simulink model "test_motion_controller"  (R2025b)
settings: Solver=FixedStepAuto  StartTime=0.0  StopTime=60  RelTol=1e-3
model workspace (MAT data in the model file):
  AmcbldcInitConf = Simulink.Parameter
  AmcbldcInitConf.Value.thresholds.jntVelMax = 40000
  AmcbldcInitConf.Value.thresholds.motorNominalCurrents = 0.34999999404
  AmcbldcInitConf.Value.thresholds.motorPeakCurrents = 0.699999988079
  AmcbldcInitConf.Value.thresholds.motorOverloadCurrents = 1
  AmcbldcInitConf.Value.thresholds.motorPwmLimit = 32000
  AmcbldcInitConf.Value.thresholds.motorCriticalTemperature = 0
  AmcbldcInitConf.Value.pids.currentPID.type : enumeration (value not decoded)
  AmcbldcInitConf.Value.pids.currentPID.OutMax = 0
  AmcbldcInitConf.Value.pids.currentPID.OutMin = 0
  AmcbldcInitConf.Value.pids.currentPID.P = 2
  AmcbldcInitConf.Value.pids.currentPID.I = 500
  AmcbldcInitConf.Value.pids.currentPID.D = 0
  AmcbldcInitConf.Value.pids.currentPID.N = 10
  AmcbldcInitConf.Value.pids.currentPID.I0 = 0
  AmcbldcInitConf.Value.pids.currentPID.D0 = 0
  AmcbldcInitConf.Value.pids.currentPID.shift_factor = 0
  AmcbldcInitConf.Value.pids.velocityPID.type : enumeration (value not decoded)
  AmcbldcInitConf.Value.pids.velocityPID.OutMax = 0
  AmcbldcInitConf.Value.pids.velocityPID.OutMin = 0
  AmcbldcInitConf.Value.pids.velocityPID.P = -20
  AmcbldcInitConf.Value.pids.velocityPID.I = -20
  AmcbldcInitConf.Value.pids.velocityPID.D = 0
  AmcbldcInitConf.Value.pids.velocityPID.N = 100
  AmcbldcInitConf.Value.pids.velocityPID.I0 = 0
  AmcbldcInitConf.Value.pids.velocityPID.D0 = 0
  AmcbldcInitConf.Value.pids.velocityPID.shift_factor = 10
  AmcbldcInitConf.Value.pids.positionPID.type : enumeration (value not decoded)
  AmcbldcInitConf.Value.pids.positionPID.OutMax = 0
  AmcbldcInitConf.Value.pids.positionPID.OutMin = 0
  AmcbldcInitConf.Value.pids.positionPID.P = 0
  AmcbldcInitConf.Value.pids.positionPID.I = 0
  AmcbldcInitConf.Value.pids.positionPID.D = 0
  AmcbldcInitConf.Value.pids.positionPID.N = 0
  AmcbldcInitConf.Value.pids.positionPID.I0 = 0
  AmcbldcInitConf.Value.pids.positionPID.D0 = 0
  AmcbldcInitConf.Value.pids.positionPID.shift_factor = 0
  AmcbldcInitConf.Value.motor.externals.enable_verbosity = 0
  AmcbldcInitConf.Value.motor.externals.has_hall_sens = 1
  AmcbldcInitConf.Value.motor.externals.has_quadrature_encoder = 0
  AmcbldcInitConf.Value.motor.externals.has_speed_quadrature_encoder = 0
  AmcbldcInitConf.Value.motor.externals.has_temperature_sens = 0
  AmcbldcInitConf.Value.motor.externals.encoder_tolerance = 0
  AmcbldcInitConf.Value.motor.externals.pole_pairs = 7
  AmcbldcInitConf.Value.motor.externals.rotor_encoder_resolution = 0
  AmcbldcInitConf.Value.motor.externals.rotor_index_offset = 0
  AmcbldcInitConf.Value.motor.externals.use_index = 0
  AmcbldcInitConf.Value.motor.Kbemf = 0
  AmcbldcInitConf.Value.motor.Rphase = 0
  AmcbldcInitConf.Value.motor.Imin = 0
  AmcbldcInitConf.Value.motor.Imax = 0
  AmcbldcInitConf.Value.motor.Vmax = 24
  AmcbldcInitConf.Value.motor.resistance = 25.8999996185
  AmcbldcInitConf.Value.motor.inductance = 271
  AmcbldcInitConf.Value.motor.thermal_resistance = 16
  AmcbldcInitConf.Value.motor.thermal_time_constant = 797.5
  AmcbldcInitConf.Value.motor.hall_sensors_offset = 30
  AmcbldcInitConf.Value.motor.hall_sensors_swapBC = 0
  AmcbldcInitConf.Value.motor.reference_encoder : enumeration (value not decoded)
  AmcbldcInitConf.Complexity = 'real'
  AmcbldcInitConf.Dimensions = [1 1]
  AmcbldcInitConf.CoderInfo.StorageClass = 'ExportedGlobal'
  AmcbldcInitConf.CoderInfo.Alias = 'AmcbldcInitConf'
  AmcbldcInitConf.DataType = 'Bus: ActuatorConfiguration'
undefined symbols (not defined in the file): ControlModes, EventTypes, MCMotorParamsSet
settings Model: DataDictionary=embeddedBoard_common.sldd  Creator=mfussi  LastModifiedBy=mfussi
settings SolverCC: ConcurrentTasks=on  AutoInsertRateTranBlk=on
settings DataIOCC: SaveOutput=off  DSMLogging=off  SaveTime=off
settings OptimizationCC: DefaultParameterBehavior=Inlined  EnhancedBackFolding=on  PassReuseOutputArgsAs=Individual arguments  ZeroExternalMemoryAtStartup=off  ZeroInternalMemoryAtStartup=off  SimCompilerOptimization=on  OptimizeBlockOrder=speed  DifferentSizesBufferReuse=on  OptimizationCustomize=off  EfficientTunableParamExpr=on
settings DebuggingCC: ParameterPrecisionLossMsg=none  ParameterTunabilityLossMsg=error
settings ModelReferenceCC: SupportModelReferenceSimTargetCustomCode=on
settings SFSimCC: MATLABDynamicMemAlloc=off  SimTargetLang=C++  SimDLTargetLibrary=mkl-dnn
settings RTWCC: SystemTargetFile=ert.tlc  TemplateMakefile=ert_default_tmf  GPUComputeCapability=3.5  Description=Embedded Coder
settings CodeAppCC: ForceParamTrailComments=on  IgnoreCustomStorageClasses=off  MaxIdLength=95.0  OperatorAnnotations=on  SimulinkDataObjDesc=on  SFDataObjDesc=on  InsertBlockDesc=on
settings ERTTargetCC: ERTCustomFileTemplate=example_file_process.tlc  TargetLangStandard=C99 (ISO)  GenerateSampleERTMain=on

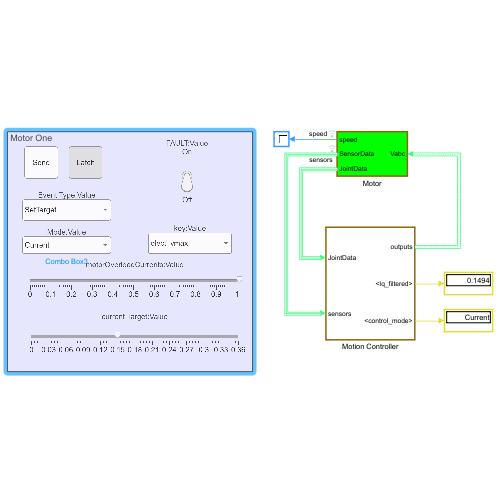
[thumbnail: Simulink's stored preview of the top-level diagram]
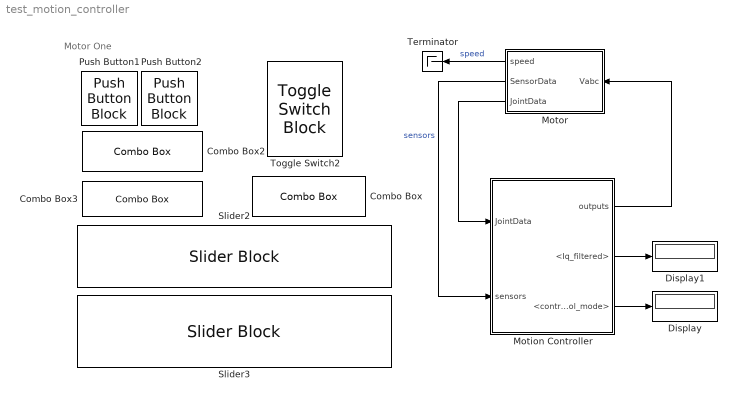
== system test_motion_controller ==
  note: Motor One
  Combo Box : ComboBox  SelectedLabel=elect_vmax  UseEnumeratedDataType=on  EnumeratedDataType=MCMotorParamsSet
  Combo Box2 : ComboBox  SelectedLabel=SetTarget  UseEnumeratedDataType=on  EnumeratedDataType=EventTypes
  Combo Box3 : ComboBox  SelectedLabel=Current  UseEnumeratedDataType=on  EnumeratedDataType=ControlModes
  Display : Display
  Display1 : Display
  Motion Controller : Subsystem
  Motor : Subsystem
  Push Button1 : PushButtonBlock  ButtonText=Send  IconOnColor=[0.0, 0.39215686274509803, 0.0]  IconOffColor=[0.0, 1.0, 0.0]  OffValue=0.000000
  Push Button2 : PushButtonBlock  ButtonText=Latch  ButtonType=Latch  IconOnColor=[0.0, 0.39215686274509803, 0.0]  IconOffColor=[0.0, 1.0, 0.0]  OffValue=0.000000
  Slider2 : SliderBlock  ScaleMax=1
  Slider3 : SliderBlock  ScaleMax=0.36
  Terminator : Terminator
  Toggle Switch2 : ToggleSwitchBlock
  wires:
  Motor/1(speed) -> Terminator/1  "speed"
  Motor/2(SensorData) -> Motion Controller/2(sensors)  "sensors"
  Motor/3(JointData) -> Motion Controller/1(JointData)
  Motion Controller/1(outputs) -> Motor/1(Vabc)
  Motion Controller/2(<Iq_filtered>) -> Display1/1
  Motion Controller/3(<control_mode>) -> Display/1

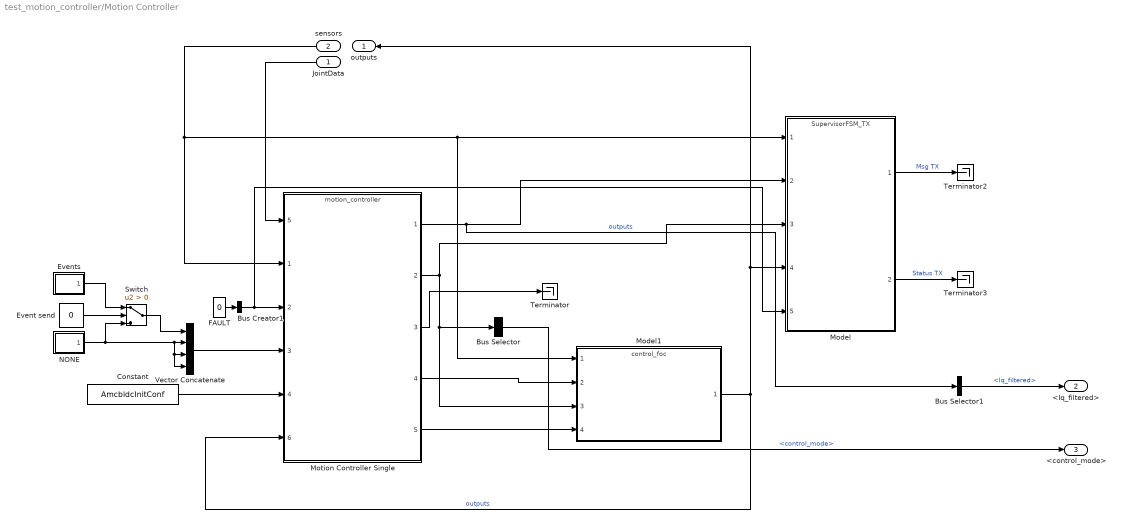
== system test_motion_controller/Motion Controller ==
  JointData : Inport
  sensors : Inport  Port=2
  Bus Creator1 : BusCreator  Inputs=1  OutDataTypeStr=Bus: ExternalFlags  NonVirtualBus=on
      settings: InheritFromInputs=off
  Bus Selector : BusSelector  OutputSignals=control_mode
  Bus Selector1 : BusSelector  OutputSignals=Iq_filtered
  Constant : Constant  Value=AmcbldcInitConf  OutDataTypeStr=Bus: ActuatorConfiguration  SampleTime=1e-3
  Event send : Constant  Value=0  OutDataTypeStr=boolean  SampleTime=1e-3
  Events : Subsystem
  FAULT : Constant  Value=0  OutDataTypeStr=Inherit: Inherit via back propagation  SampleTime=0.001
  Model : ModelReference  ModelNameDialog=SupervisorFSM_TX.slx  SimulationMode=Normal  ModelReferenceVersion=11.18
  Model1 : ModelReference  ModelNameDialog=control_foc.slx  SimulationMode=Normal  ModelReferenceVersion=10.10
  Motion Controller Single : ModelReference  ModelNameDialog=motion_controller.slx  ModelReferenceVersion=6.14
      settings: PortSchema="{\"entries\":[{\"content\":{\"sides\":[{\"content\":{\"connectorIds\":[\"In5\",\"In1\",\"In2\",\"In3\",\"In4\",\"In6\"]},\"type\":\"ConnectorPlacement.EquallySpacedRectSide\",\"uuid\":\"3236986d-16bb-4c67-8dea-b6bfcbd43a75\"},{\"content\":{\"connectorIds\":[\"Out1\",\"Out2\",\"Out3\",\"Out4\",\"Out5\"],\"side\":\"RIGHT\"},\"type\":\"ConnectorPlacement.EquallySpacedRectSide\",\"uuid\":\"7377f631-7d64-4109-b716-f3a651661c1a\"},{\"content\":{\"side\":\"TOP\"},\"type\":\"ConnectorPlacement.EquallySpacedRectSide\",\"uuid\":\"dfb06a46-8687-4228-b411-547df7d03d54\"}]},\"type\":\"ConnectorPlacement.EquallySpacedConnector\",\"uuid\":\"7aeaa35f-2805-4a8c-90e3-68b95f5da4bc\"}],\"packageUris\":[\"http://schema.mathworks.com/mf0/Connector/R2020b\"],\"version\":\"1.0\"}"
  NONE : Subsystem
  Switch : Switch  Criteria=u2 > Threshold  SaturateOnIntegerOverflow=off  InputSameDT=off
  Terminator : Terminator
  Terminator2 : Terminator
  Terminator3 : Terminator
  Vector Concatenate : Concatenate  NumInputs=4
  outputs : Outport
  <Iq_filtered> : Outport  Port=2
  <control_mode> : Outport  Port=3
  wires:
  Bus Creator1/1 -> Model/5, Motion Controller Single/2
  sensors/1 -> Model/1, Model1/1, Motion Controller Single/1
  Switch/1 -> Vector Concatenate/1
  Model/2 -> Terminator3/1  "Status TX"
  Event send/1 -> Switch/2
  Motion Controller Single/1 -> Bus Selector1/1, Model/2  "outputs"
  Constant/1 -> Motion Controller Single/4
  Model/1 -> Terminator2/1  "Msg TX"
  Model1/1 -> Motion Controller Single/6, outputs/1, Model/4  "outputs"
  Motion Controller Single/2 -> Bus Selector/1, Model1/3, Model/3
  JointData/1 -> Motion Controller Single/5
  Events/1(Events) -> Switch/1
  FAULT/1 -> Bus Creator1/1
  Motion Controller Single/4 -> Model1/2
  NONE/1(Events) -> Switch/3, Vector Concatenate/3, Vector Concatenate/4, Vector Concatenate/2
  Motion Controller Single/5 -> Model1/4
  Bus Selector1/1 -> <Iq_filtered>/1  "<Iq_filtered>"
  Vector Concatenate/1 -> Motion Controller Single/3
  Motion Controller Single/3 -> Terminator/1
  Bus Selector/1 -> <control_mode>/1  "<control_mode>"

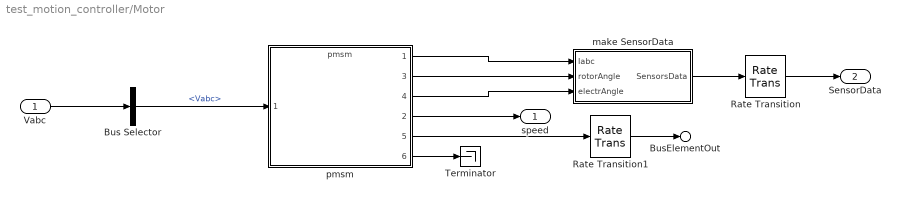
== system test_motion_controller/Motor ==
  Vabc : Inport
  Bus Selector : BusSelector  OutputSignals=Vabc
  Rate Transition : RateTransition  Integrity=off  OutPortSampleTime=Ts_ControlFOC
  Rate Transition1 : RateTransition  Integrity=off  OutPortSampleTime=Ts_ControlFOC
  Terminator : Terminator
  make SensorData : Subsystem
  pmsm : ModelReference  ModelNameDialog=pmsm.slx  SimulationMode=Normal  ModelReferenceVersion=11.7
      settings: PortSchema="{\"entries\":[{\"content\":{\"sides\":[{\"content\":{\"connectorIds\":[\"In1\"]},\"type\":\"ConnectorPlacement.EquallySpacedRectSide\",\"uuid\":\"8cec65a8-4219-41d1-959d-4e8d996cc561\"},{\"content\":{\"connectorIds\":[\"Out1\",\"Out3\",\"Out4\",\"Out2\",\"Out5\",\"Out6\"],\"side\":\"RIGHT\"},\"type\":\"ConnectorPlacement.EquallySpacedRectSide\",\"uuid\":\"120dfdfb-4ec8-4266-9e58-5a4f10fe78d1\"},{\"content\":{\"side\":\"TOP\"},\"type\":\"ConnectorPlacement.EquallySpacedRectSide\",\"uuid\":\"6d35c191-eb3f-4663-84d3-c95352a14c82\"}]},\"type\":\"ConnectorPlacement.EquallySpacedConnector\",\"uuid\":\"bf10708e-bbfb-4369-9195-0995d9345086\"}],\"packageUris\":[\"http://schema.mathworks.com/mf0/Connector/R2020b\"],\"version\":\"1.0\"}"
  speed : Outport
  SensorData : Outport  Port=2  OutDataTypeStr=Bus: SensorsData
  BusElementOut : Outport  Description=position encoder after gearbox  Port=3  PortName=JointData  Element=position
  wires:
  make SensorData/1(SensorsData) -> Rate Transition/1
  pmsm/1 -> make SensorData/1(Iabc)
  Bus Selector/1 -> pmsm/1  "<Vabc>"
  Vabc/1 -> Bus Selector/1
  Rate Transition/1 -> SensorData/1
  pmsm/4 -> make SensorData/3(electrAngle)
  pmsm/2 -> speed/1
  pmsm/3 -> make SensorData/2(rotorAngle)
  pmsm/5 -> Rate Transition1/1
  pmsm/6 -> Terminator/1
  Rate Transition1/1 -> BusElementOut/1

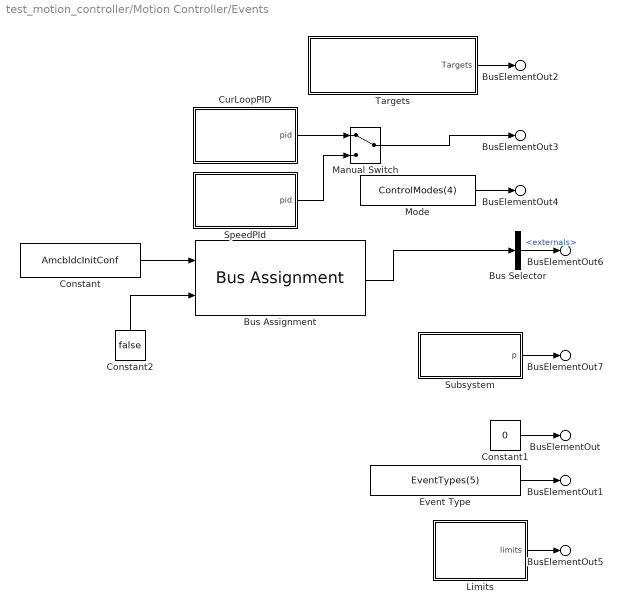
== system test_motion_controller/Motion Controller/Events ==
  Bus Assignment : BusAssignment  AssignedSignals=motor.externals.has_quadrature_encoder
  Bus Selector : BusSelector  OutputSignals=motor.externals
  Constant : Constant  Value=AmcbldcInitConf  OutDataTypeStr=Bus: ActuatorConfiguration
  Constant1 : Constant  Value=0  OutDataTypeStr=uint8
  Constant2 : Constant  Value=false  OutDataTypeStr=boolean
  CurLoopPID : Subsystem  mask{OutMax=0, OutMin=0, P=2, I=500, D=0, N=10, I0=0, D0=0, shift_factor=0}
      mask prompts: shift_factor "Shift Factor"
  Event Type : Constant  Value=EventTypes(5)  OutDataTypeStr=Enum: EventTypes
  Limits : Subsystem
  Manual Switch : ManualSwitch
  Mode : Constant  Value=ControlModes(4)  OutDataTypeStr=Enum: ControlModes
  SpeedPId : Subsystem  mask{OutMax=0, OutMin=0, P=1e-5, I=1e-4, D=0, N=0, I0=0, D0=0, shift_factor=0}
      mask prompts: shift_factor "Shift Factor"
  Subsystem : Subsystem
  Targets : Subsystem
  BusElementOut : Outport  PortName=Events  Element=motor_id
  BusElementOut1 : Outport  PortName=Events  Element=event_type
  BusElementOut2 : Outport  PortName=Events  Element=targets_content
  BusElementOut3 : Outport  PortName=Events  Element=pid_content
  BusElementOut4 : Outport  PortName=Events  Element=control_mode_content
  BusElementOut5 : Outport  PortName=Events  Element=limits_content
  BusElementOut6 : Outport  PortName=Events  Element=motor_config_content
  BusElementOut7 : Outport  PortName=Events  Element=motor_config_set
  wires:
  Targets/1(Targets) -> BusElementOut2/1
  Mode/1 -> BusElementOut4/1
  Manual Switch/1 -> BusElementOut3/1
  Bus Assignment/1 -> Bus Selector/1
  Constant1/1 -> BusElementOut/1
  Limits/1("limits ") -> BusElementOut5/1
  Event Type/1 -> BusElementOut1/1
  Bus Selector/1 -> BusElementOut6/1  "<externals>"
  CurLoopPID/1(pid) -> Manual Switch/1
  SpeedPId/1(pid) -> Manual Switch/2
  Constant/1 -> Bus Assignment/1
  Constant2/1 -> Bus Assignment/2
  Subsystem/1(p) -> BusElementOut7/1

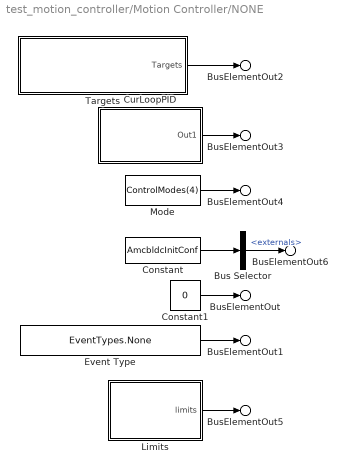
== system test_motion_controller/Motion Controller/NONE ==
  Bus Selector : BusSelector  OutputSignals=motor.externals
  Constant : Constant  Value=AmcbldcInitConf  OutDataTypeStr=Bus: ActuatorConfiguration
  Constant1 : Constant  Value=0  OutDataTypeStr=uint8
  CurLoopPID : Subsystem  mask{OutMax=0, OutMin=0, P=20, I=5000, D=0, N=10, I0=0, D0=0, shift_factor=0}
      mask prompts: shift_factor "Shift Factor"
  Event Type : Constant  Value=EventTypes.None  OutDataTypeStr=Enum: EventTypes
  Limits : Subsystem
  Mode : Constant  Value=ControlModes(4)  OutDataTypeStr=Enum: ControlModes
  Targets : Subsystem
  BusElementOut : Outport  PortName=Events  Element=motor_id
  BusElementOut1 : Outport  PortName=Events  Element=event_type
  BusElementOut2 : Outport  PortName=Events  Element=targets_content
  BusElementOut3 : Outport  PortName=Events  Element=pid_content
  BusElementOut4 : Outport  PortName=Events  Element=control_mode_content
  BusElementOut5 : Outport  PortName=Events  Element=limits_content
  BusElementOut6 : Outport  PortName=Events  Element=motor_config_content
  wires:
  Targets/1(Targets) -> BusElementOut2/1
  CurLoopPID/1(Out1) -> BusElementOut3/1
  Bus Selector/1 -> BusElementOut6/1  "<externals>"
  Limits/1("limits ") -> BusElementOut5/1
  Constant/1 -> Bus Selector/1
  Mode/1 -> BusElementOut4/1
  Constant1/1 -> BusElementOut/1
  Event Type/1 -> BusElementOut1/1

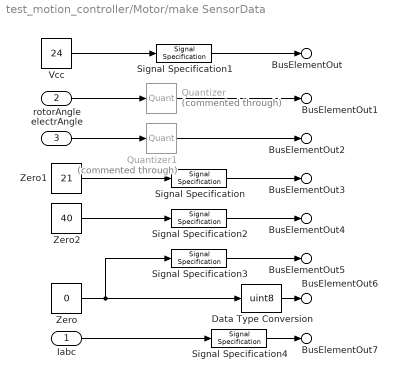
== system test_motion_controller/Motor/make SensorData ==
  Iabc : Inport
  rotorAngle : Inport  Port=2
  electrAngle : Inport  Port=3
  Data Type Conversion : DataTypeConversion  OutDataTypeStr=uint8  SaturateOnIntegerOverflow=off  RndMeth=Floor
  Quantizer : Quantizer  Commented=through  QuantizationInterval=60
  Quantizer1 : Quantizer  Commented=through  QuantizationInterval=60
  Signal Specification : SignalSpecification  Unit=degC
  Signal Specification1 : SignalSpecification  Unit=V
  Signal Specification2 : SignalSpecification  Unit=V
  Signal Specification3 : SignalSpecification  Unit=A
  Signal Specification4 : SignalSpecification  Unit=A
  Vcc : Constant  Value=24  OutDataTypeStr=single
  Zero : Constant  Value=0  OutDataTypeStr=single
  Zero1 : Constant  Value=21  OutDataTypeStr=single
  Zero2 : Constant  Value=40  OutDataTypeStr=single
  BusElementOut : Outport  Description=power supply voltage  PortName=SensorsData  Element=driversensors.Vcc
  BusElementOut1 : Outport  Description=Mechanical Angle before gearbox  PortName=SensorsData  Element=motorsensors.qencoder.rotor_angle
  BusElementOut7 : Outport  PortName=SensorsData  Element=motorsensors.Iabc
  BusElementOut2 : Outport  Description=electrical angle = angle * pole_pairs  PortName=SensorsData  Element=motorsensors.electrical_angle
  BusElementOut3 : Outport  PortName=SensorsData  Element=motorsensors.temperature
  BusElementOut4 : Outport  PortName=SensorsData  Element=motorsensors.voltage
  BusElementOut5 : Outport  PortName=SensorsData  Element=motorsensors.current
  BusElementOut6 : Outport  PortName=SensorsData  Element=motorsensors.hallABC
  wires:
  rotorAngle/1 -> Quantizer/1
  electrAngle/1 -> Quantizer1/1
  Vcc/1 -> Signal Specification1/1
  Quantizer1/1 -> BusElementOut2/1
  Iabc/1 -> Signal Specification4/1
  Quantizer/1 -> BusElementOut1/1
  Data Type Conversion/1 -> BusElementOut6/1
  Signal Specification/1 -> BusElementOut3/1
  Signal Specification3/1 -> BusElementOut5/1
  Signal Specification2/1 -> BusElementOut4/1
  Signal Specification1/1 -> BusElementOut/1
  Signal Specification4/1 -> BusElementOut7/1
  Zero/1 -> Signal Specification3/1, Data Type Conversion/1
  Zero1/1 -> Signal Specification/1
  Zero2/1 -> Signal Specification2/1

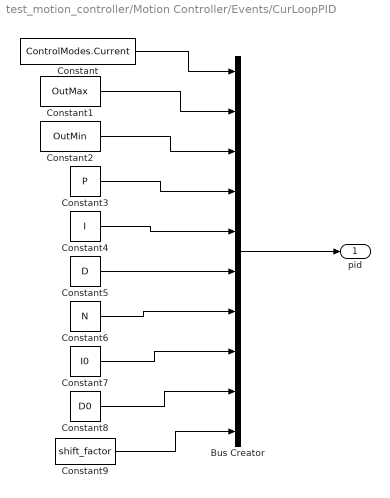
== system test_motion_controller/Motion Controller/Events/CurLoopPID ==
  Bus Creator : BusCreator  Inputs=10  OutDataTypeStr=Bus: PID  NonVirtualBus=on
      settings: InheritFromInputs=off
  Constant : Constant  Value=ControlModes.Current
  Constant1 : Constant  Value=OutMax  OutDataTypeStr=single
  Constant2 : Constant  Value=OutMin  OutDataTypeStr=single
  Constant3 : Constant  Value=P  OutDataTypeStr=single
  Constant4 : Constant  Value=I  OutDataTypeStr=single
  Constant5 : Constant  Value=D  OutDataTypeStr=single
  Constant6 : Constant  Value=N  OutDataTypeStr=single
  Constant7 : Constant  Value=I0  OutDataTypeStr=single
  Constant8 : Constant  Value=D0  OutDataTypeStr=single
  Constant9 : Constant  Value=shift_factor  OutDataTypeStr=uint8
  pid : Outport  OutDataTypeStr=Bus: PID
  wires:
  Bus Creator/1 -> pid/1
  Constant8/1 -> Bus Creator/9
  Constant3/1 -> Bus Creator/4
  Constant5/1 -> Bus Creator/6
  Constant1/1 -> Bus Creator/2
  Constant7/1 -> Bus Creator/8
  Constant2/1 -> Bus Creator/3
  Constant9/1 -> Bus Creator/10
  Constant4/1 -> Bus Creator/5
  Constant/1 -> Bus Creator/1
  Constant6/1 -> Bus Creator/7

== system test_motion_controller/Motion Controller/Events/Limits ==
  Bus Creator : BusCreator  Inputs=4  OutDataTypeStr=Bus: SupervisorInputLimits  NonVirtualBus=on
      settings: InheritFromInputs=off
  Constant2 : Constant  Value=ControlModes.Current  OutDataTypeStr=Enum: ControlModes
  motorNominalCurrents : Constant  Value=5  OutDataTypeStr=single
  motorOverloadCurrents : Constant  Value=10  OutDataTypeStr=single
  motorPeakCurrents : Constant  Value=5  OutDataTypeStr=single
  "limits " : Outport
  wires:
  motorNominalCurrents/1 -> Bus Creator/2
  Constant2/1 -> Bus Creator/4
  motorOverloadCurrents/1 -> Bus Creator/1
  motorPeakCurrents/1 -> Bus Creator/3
  Bus Creator/1 -> "limits "/1

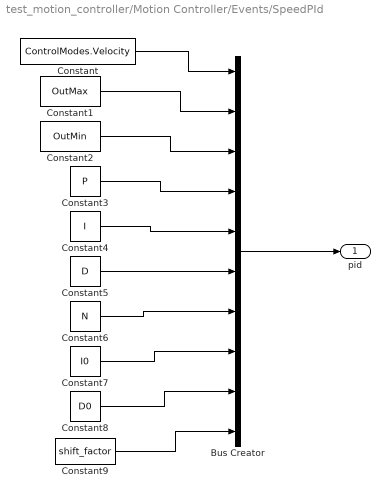
== system test_motion_controller/Motion Controller/Events/SpeedPId ==
  Bus Creator : BusCreator  Inputs=10  OutDataTypeStr=Bus: PID  NonVirtualBus=on
      settings: InheritFromInputs=off
  Constant : Constant  Value=ControlModes.Velocity
  Constant1 : Constant  Value=OutMax  OutDataTypeStr=single
  Constant2 : Constant  Value=OutMin  OutDataTypeStr=single
  Constant3 : Constant  Value=P  OutDataTypeStr=single
  Constant4 : Constant  Value=I  OutDataTypeStr=single
  Constant5 : Constant  Value=D  OutDataTypeStr=single
  Constant6 : Constant  Value=N  OutDataTypeStr=single
  Constant7 : Constant  Value=I0  OutDataTypeStr=single
  Constant8 : Constant  Value=D0  OutDataTypeStr=single
  Constant9 : Constant  Value=shift_factor  OutDataTypeStr=uint8
  pid : Outport  OutDataTypeStr=Bus: PID
  wires:
  Bus Creator/1 -> pid/1
  Constant8/1 -> Bus Creator/9
  Constant3/1 -> Bus Creator/4
  Constant5/1 -> Bus Creator/6
  Constant1/1 -> Bus Creator/2
  Constant7/1 -> Bus Creator/8
  Constant2/1 -> Bus Creator/3
  Constant9/1 -> Bus Creator/10
  Constant4/1 -> Bus Creator/5
  Constant/1 -> Bus Creator/1
  Constant6/1 -> Bus Creator/7

== system test_motion_controller/Motion Controller/Events/Subsystem ==
  Select motor param : Subsystem
  Vmax : Constant  Value=40  OutDataTypeStr=single
  hall offset : Constant  Value=30  OutDataTypeStr=single
  hall swap mode : Constant  OutDataTypeStr=single
  kbemf : Constant  Value=0.032  OutDataTypeStr=single
  p : Outport
  wires:
  Select motor param/1(param_set) -> p/1
  hall swap mode/1 -> Select motor param/3(hall swap mode)
  Vmax/1 -> Select motor param/4(Vmax)
  hall offset/1 -> Select motor param/2(hall offset)
  kbemf/1 -> Select motor param/1(kbemf)

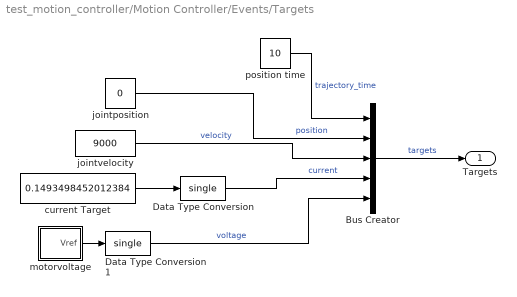
== system test_motion_controller/Motion Controller/Events/Targets ==
  Bus Creator : BusCreator  Inputs=5  OutDataTypeStr=Bus: Targets  NonVirtualBus=on
  Data Type Conversion : DataTypeConversion  OutDataTypeStr=single  SaturateOnIntegerOverflow=off  RndMeth=Floor
  Data Type Conversion1 : DataTypeConversion  OutDataTypeStr=single  SaturateOnIntegerOverflow=off  RndMeth=Floor
  current Target : Constant  Value=0.1493498452012384
  jointposition : Constant  Value=0  OutDataTypeStr=single
  jointvelocity : Constant  Value=9000  OutDataTypeStr=single
  motorvoltage : Subsystem
  position time : Constant  Value=10  OutDataTypeStr=single
  Targets : Outport
  wires:
  Bus Creator/1 -> Targets/1  "targets"
  jointposition/1 -> Bus Creator/2  "position"
  jointvelocity/1 -> Bus Creator/3  "velocity"
  Data Type Conversion1/1 -> Bus Creator/5  "voltage"
  Data Type Conversion/1 -> Bus Creator/4  "current"
  motorvoltage/1(Vref) -> Data Type Conversion1/1
  current Target/1 -> Data Type Conversion/1
  position time/1 -> Bus Creator/1  "trajectory_time"

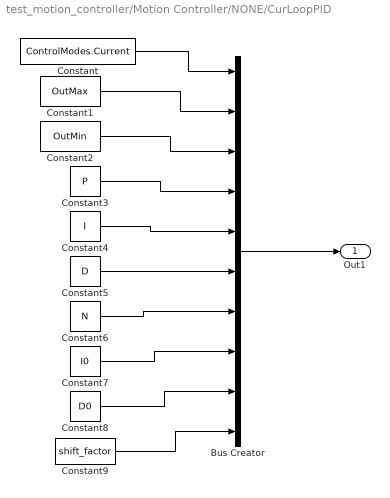
== system test_motion_controller/Motion Controller/NONE/CurLoopPID ==
  Bus Creator : BusCreator  Inputs=10  OutDataTypeStr=Bus: PID  NonVirtualBus=on
      settings: InheritFromInputs=off
  Constant : Constant  Value=ControlModes.Current
  Constant1 : Constant  Value=OutMax  OutDataTypeStr=single
  Constant2 : Constant  Value=OutMin  OutDataTypeStr=single
  Constant3 : Constant  Value=P  OutDataTypeStr=single
  Constant4 : Constant  Value=I  OutDataTypeStr=single
  Constant5 : Constant  Value=D  OutDataTypeStr=single
  Constant6 : Constant  Value=N  OutDataTypeStr=single
  Constant7 : Constant  Value=I0  OutDataTypeStr=single
  Constant8 : Constant  Value=D0  OutDataTypeStr=single
  Constant9 : Constant  Value=shift_factor  OutDataTypeStr=uint8
  Out1 : Outport  OutDataTypeStr=Bus: PID
  wires:
  Bus Creator/1 -> Out1/1
  Constant8/1 -> Bus Creator/9
  Constant3/1 -> Bus Creator/4
  Constant5/1 -> Bus Creator/6
  Constant1/1 -> Bus Creator/2
  Constant7/1 -> Bus Creator/8
  Constant2/1 -> Bus Creator/3
  Constant9/1 -> Bus Creator/10
  Constant4/1 -> Bus Creator/5
  Constant/1 -> Bus Creator/1
  Constant6/1 -> Bus Creator/7

== system test_motion_controller/Motion Controller/NONE/Limits ==
  Bus Creator : BusCreator  Inputs=4  OutDataTypeStr=Bus: SupervisorInputLimits  NonVirtualBus=on
      settings: InheritFromInputs=off
  Constant2 : Constant  Value=ControlModes.Current  OutDataTypeStr=Enum: ControlModes
  motorNominalCurrents : Constant  Value=0.7  OutDataTypeStr=single
  motorOverloadCurrents : Constant  Value=0.8730650154798761  OutDataTypeStr=single
  motorPeakCurrents : Constant  Value=0.7  OutDataTypeStr=single
  "limits " : Outport
  wires:
  motorNominalCurrents/1 -> Bus Creator/2
  Constant2/1 -> Bus Creator/4
  motorOverloadCurrents/1 -> Bus Creator/1
  motorPeakCurrents/1 -> Bus Creator/3
  Bus Creator/1 -> "limits "/1

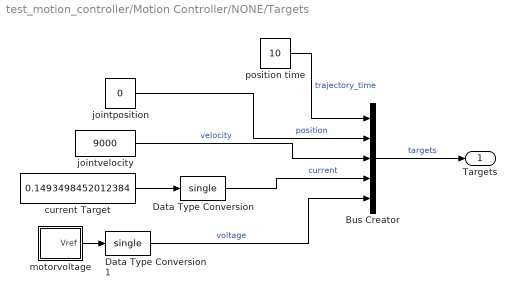
== system test_motion_controller/Motion Controller/NONE/Targets ==
  Bus Creator : BusCreator  Inputs=5  OutDataTypeStr=Bus: Targets  NonVirtualBus=on
  Data Type Conversion : DataTypeConversion  OutDataTypeStr=single  SaturateOnIntegerOverflow=off  RndMeth=Floor
  Data Type Conversion1 : DataTypeConversion  OutDataTypeStr=single  SaturateOnIntegerOverflow=off  RndMeth=Floor
  current Target : Constant  Value=0.1493498452012384
  jointposition : Constant  Value=0  OutDataTypeStr=single
  jointvelocity : Constant  Value=9000  OutDataTypeStr=single
  motorvoltage : Subsystem
  position time : Constant  Value=10  OutDataTypeStr=single
  Targets : Outport
  wires:
  Bus Creator/1 -> Targets/1  "targets"
  jointposition/1 -> Bus Creator/2  "position"
  jointvelocity/1 -> Bus Creator/3  "velocity"
  Data Type Conversion1/1 -> Bus Creator/5  "voltage"
  Data Type Conversion/1 -> Bus Creator/4  "current"
  motorvoltage/1(Vref) -> Data Type Conversion1/1
  current Target/1 -> Data Type Conversion/1
  position time/1 -> Bus Creator/1  "trajectory_time"

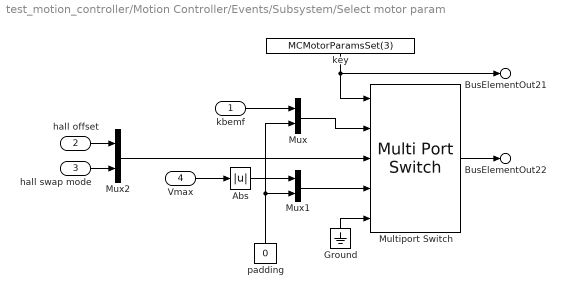
== system test_motion_controller/Motion Controller/Events/Subsystem/Select motor param ==
  kbemf : Inport
  hall offset : Inport  Port=2
  hall swap mode : Inport  Port=3
  Vmax : Inport  Port=4  OutDataTypeStr=single
  Abs : Abs  SaturateOnIntegerOverflow=off
  Ground : Ground
  Multiport Switch : MultiPortSwitch  DataPortOrder=Specify indices  DataPortIndices={MCMotorParamsSet.Kbemf, MCMotorParamsSet.hall, MCMotorParamsSet.elect_vmax}  DataPortForDefault=Additional data port  DiagnosticForDefault=None  SaturateOnIntegerOverflow=off  InputSameDT=off
  Mux : Mux  Inputs=2
  Mux1 : Mux  Inputs=2
  Mux2 : Mux  Inputs=2
  key : Constant  Value=MCMotorParamsSet(3)  OutDataTypeStr=Enum: MCMotorParamsSet
  padding : Constant  Value=0  OutDataTypeStr=single
  BusElementOut21 : Outport  PortName=param_set  Element=key
  BusElementOut22 : Outport  PortName=param_set  Element=value
  wires:
  Mux/1 -> Multiport Switch/2
  kbemf/1 -> Mux/1
  Mux2/1 -> Multiport Switch/3
  Mux1/1 -> Multiport Switch/4
  Ground/1 -> Multiport Switch/5
  padding/1 -> Mux/2, Mux1/2
  hall offset/1 -> Mux2/1
  hall swap mode/1 -> Mux2/2
  Vmax/1 -> Abs/1
  key/1 -> BusElementOut21/1, Multiport Switch/1
  Multiport Switch/1 -> BusElementOut22/1
  Abs/1 -> Mux1/1

== system test_motion_controller/Motion Controller/Events/Targets/motorvoltage ==
  Constant : Constant  Value=20
  Sum : Sum  Inputs=|+-
  Vref : Outport
  wires:
  Sum/1 -> Vref/1
  Constant/1 -> Sum/1

== system test_motion_controller/Motion Controller/NONE/Targets/motorvoltage ==
  Constant : Constant  Value=20
  Sum : Sum  Inputs=|+-
  Vref : Outport
  wires:
  Sum/1 -> Vref/1
  Constant/1 -> Sum/1
